simulink subsystem "FourActuatorAWD"  (R2024a)
settings: Solver=VariableStepAuto  StartTime=0.0  StopTime=10.0  RelTol=1e-3
settings Model: Creator=The MathWorks, Inc.  LastModifiedBy=The MathWorks, Inc.
settings OptimizationCC: ReuseModelBlockBuffer=off
settings RTWCC: GPUComputeCapability=3.5

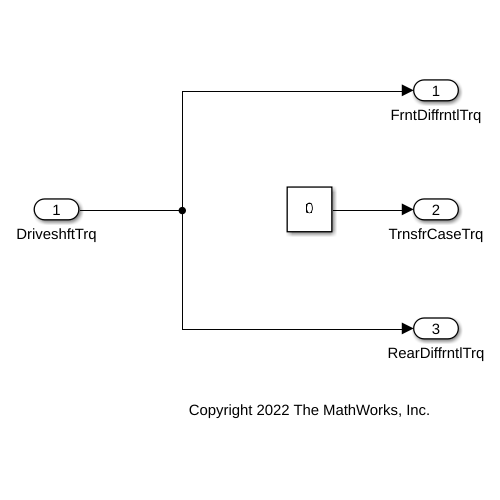
[thumbnail: Simulink's stored preview of the top-level diagram]
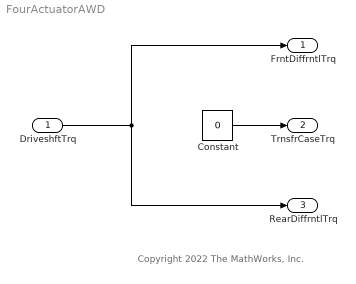
== system FourActuatorAWD ==
  note: Copyright 2022 The MathWorks, Inc.
  DriveshftTrq : Inport
  Constant : Constant  Value=0  SampleTime=-1
  FrntDiffrntlTrq : Outport
  TrnsfrCaseTrq : Outport  Port=2
  RearDiffrntlTrq : Outport  Port=3
  wires:
  DriveshftTrq/1 -> RearDiffrntlTrq/1, FrntDiffrntlTrq/1
  Constant/1 -> TrnsfrCaseTrq/1
